simulink model "mainV02_12"  (R2016b)
settings: Solver=ode23s  StartTime=0.0  StopTime=inf  MaxStep=0.2  RelTol=1e-2
undefined symbols (not defined in the file): checks, deltae_degrees, deltafl_degrees, deltafr_degrees, deltar_degrees, deltat_1, deltat_2, deltat_3, deltat_4, deltat_5, Earth, F, ft, groundReaction, initialValues, LD, Light, m, MIL, Newton, Raphson, s, WGS84
libraries: aerolibutil x8, aerolibasang x5, aerolib6dof2 x4, aerolibwind2 x3, aerolibtransform2 x3, aerolib6dofsys x3, aerolibbdyn x3, aerolibconvert2 x3, aerolibconvert x2, aerolibatmos2 x1, aerolibobsolete x1, aerolibadyn x1
(part 1 of 3)
settings Model: Creator=Uxío  LastModifiedBy=sork9
settings DataIOCC: ReturnWorkspaceOutputs=on  ReturnWorkspaceOutputsName=spidata
settings OptimizationCC: EfficientMapNaN2IntZero=off  SimCompilerOptimization=on
settings DebuggingCC: ReadBeforeWriteMsg=DisableAll  WriteAfterWriteMsg=DisableAll  WriteAfterReadMsg=DisableAll  MultiTaskDSMMsg=none
settings HardwareCC: TargetBitPerPointer=64  TargetBitPerSizeT=64  TargetBitPerPtrDiffT=64  TargetLongLongMode=on  TargetIntDivRoundTo=Zero  TargetEndianess=LittleEndian  TargetWordSize=64  TargetHWDeviceType=MATLAB Host  ProdEqTarget=off
settings ModelReferenceCC: UpdateModelReferenceTargets=IfOutOfDate
settings SFSimCC: SFSimEcho=off
settings CodeAppCC: MaxIdLength=128
settings GRTTargetCC: TargetLangStandard=C89/C90 (ANSI)  CombineOutputUpdateFcns=off  GRTInterface=on
settings ConfigComp: PSAutoStubLUT=on

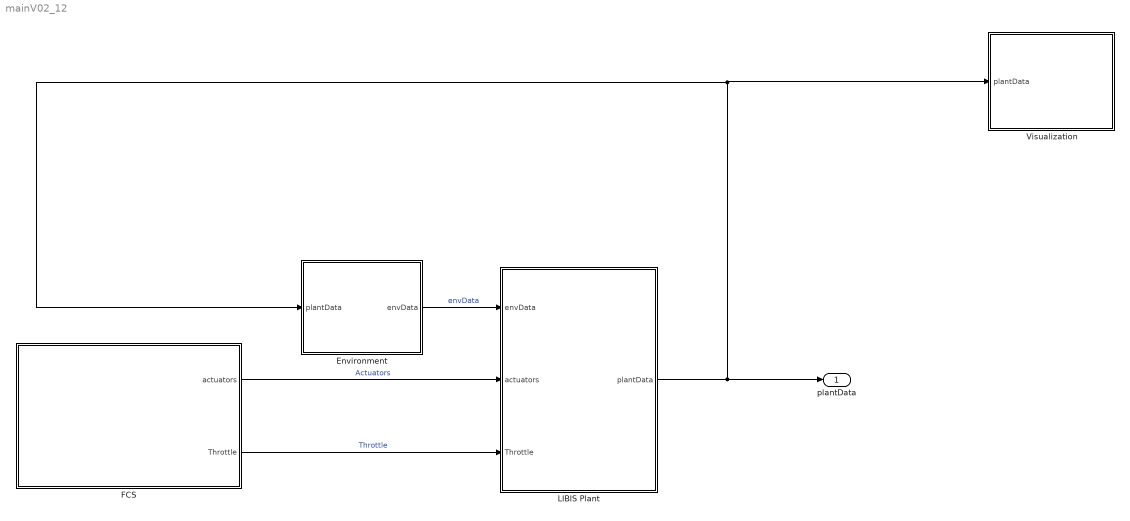
== system mainV02_12 ==
  Environment : Subsystem
      mask Display:
      | imageName='Wind.png';
      | currentPath=get_param(bdroot, 'FileName');
      | positions=strfind(currentPath,'\');
      | imagePath=strcat(currentPath(1:positions(end-1)),'graphics\',imageName);
      | image(imagePath);
  FCS : Subsystem
      mask Display:
      | imageName='FCS.png';
      | currentPath=get_param(bdroot, 'FileName');
      | positions=strfind(currentPath,'\');
      | imagePath=strcat(currentPath(1:positions(end-1)),'graphics\',imageName);
      | image(imagePath);
  LIBIS Plant : Subsystem
      mask Display:
      | imageName='LIBIS_Plant.jpg';
      | currentPath=get_param(bdroot, 'FileName');
      | positions=strfind(currentPath,'\');
      | imagePath=strcat(currentPath(1:positions(end-1)),'graphics\',imageName);
      | image(imagePath);
  Visualization : Subsystem
  plantData : Outport
  wires:
  Environment/1(envData) -> LIBIS Plant/1(envData)  "envData"
  FCS/1(actuators) -> LIBIS Plant/2(actuators)  "Actuators"
  FCS/2(Throttle) -> LIBIS Plant/3(Throttle)  "Throttle"
  LIBIS Plant/1(plantData) -> Environment/1(plantData), Visualization/1(plantData), plantData/1

== system mainV02_12/Environment ==
  plantData : Inport
  Bus Selector : BusSelector  OutputSignals=LLA.Altitude_m,X_ned,V_ned,DCM_body_earth,LLA.Latitude_deg
  COESA Atmosphere Model : aerolibatmos2/COESA Atmosphere Model  units=Metric (MKS)  spec=1976 COESA-extended U.S. Standard Atmosphere  model=Profile  profile_var=High temperature  profile_percent=1%  profile_alt=5 km (16404 ft)  envelope_var=High temperature  envelope_percent=1%  action=Warning
  Gravity in Earth Axes : Gain  Gain=[0 0 LD.Inertia.mass]  SaturateOnIntegerOverflow=on  OutDataTypeStr=Inherit: Same as input  ParamDataTypeStr=Inherit: Same as input
  Math Function : Math  Operator=transpose  SaturateOnIntegerOverflow=on
  Reshape : Reshape
  Reshape1 : Reshape
  Terrain : Subsystem
  To Body Axes : Product  Multiplication=Matrix(*)  SaturateOnIntegerOverflow=on  InputSameDT=on  OutDataTypeStr=Inherit: Same as first input
  To Body Axes1 : Product  Multiplication=Matrix(*)  SaturateOnIntegerOverflow=on  InputSameDT=on  OutDataTypeStr=Inherit: Same as first input
  WGS84 Gravity Model : aerolibobsolete/WGS84 Gravity Model  model=WGS84 Taylor Series  units=Metric (MKS)  no_atmos=on  precessing=on  month=February  day=1  year=2000  no_centrifugal=on  action=Warning
  Wind Models : Subsystem
  envDataBus : BusCreator  Inputs='h_ground','Fground','windVelocity','windOmega','T','a','P','AirDensity','Fgravity'  OutDataTypeStr=Bus: envDataBus  NonVirtualBus=on
  envData : Outport  InitialOutput=0
  wires:
  [Altitude] -> COESA Atmosphere Model/1
  Bus Selector/4 -> To Body Axes/1, Wind Models/3(DCM_be), To Body Axes1/1  "<DCM_body_earth>"
  Bus Selector/5 -> WGS84 Gravity Model/2  "<Latitude_deg>"
  Bus Selector/3 -> Wind Models/1(Ve), Terrain/2(Ve)  "<V_ned>"
  [Altitude] -> WGS84 Gravity Model/1
  envDataBus/1 -> envData/1  "envData"
  To Body Axes/1 -> Reshape/1  "Fg"
  Wind Models/2(windOmega) -> envDataBus/4  "windOmega"
  Bus Selector/2 -> Terrain/1(Xe)  "<X_ned>"
  WGS84 Gravity Model/1 -> Gravity in Earth Axes/1
  COESA Atmosphere Model/3 -> envDataBus/7  "P"
  COESA Atmosphere Model/2 -> envDataBus/6  "a"
  Wind Models/1(windVelocity) -> envDataBus/3  "windVelocity"
  [Altitude] -> Wind Models/2(Altitude)
  COESA Atmosphere Model/1 -> envDataBus/5  "T"
  COESA Atmosphere Model/4 -> envDataBus/8  "AirDensity"
  Terrain/1(hground) -> envDataBus/1  "h_ground"
  Bus Selector/1 -> [Altitude]  "<Altitude_m>"
  Gravity in Earth Axes/1 -> Math Function/1
  Math Function/1 -> To Body Axes/2
  Reshape/1 -> envDataBus/9  "Fgravity"
  To Body Axes1/1 -> Reshape1/1  "Fground_body"
  Reshape1/1 -> envDataBus/2  "Fground"
  Terrain/2(Fground) -> To Body Axes1/2  "Fground_earth"
  plantData/1 -> Bus Selector/1

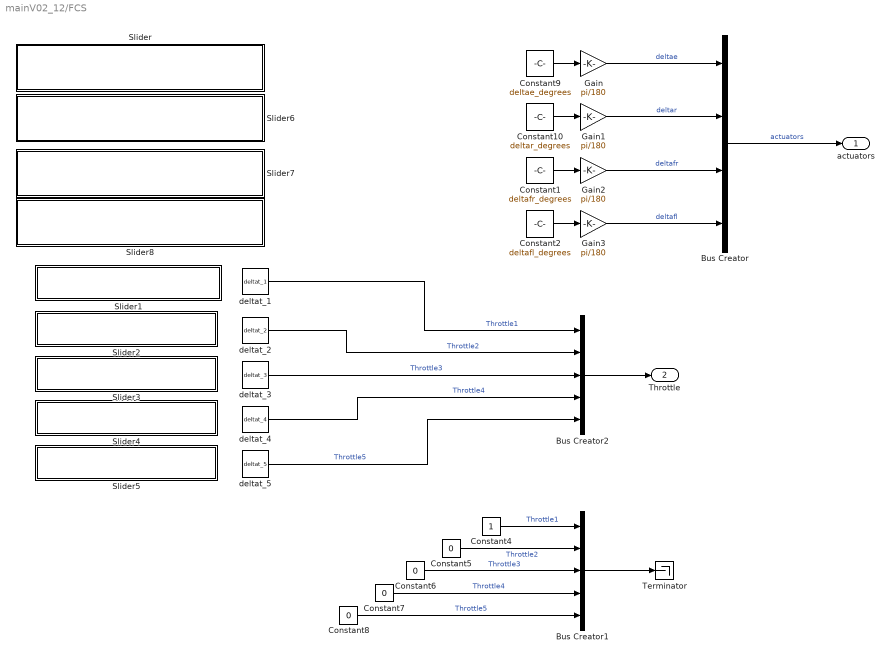
== system mainV02_12/FCS ==
  Bus Creator : BusCreator  Inputs=4
  Bus Creator1 : BusCreator  Inputs=5
  Bus Creator2 : BusCreator  Inputs=5
  Constant1 : Constant  Value=deltafr_degrees
  Constant10 : Constant  Value=deltar_degrees
  Constant2 : Constant  Value=deltafl_degrees
  Constant4 : Constant
  Constant{5..8} (4 alike) : Constant  Value=0
  Constant9 : Constant  Value=deltae_degrees
  Gain{,1..3} (4 alike) : Gain  Gain=pi/180
  Slider : Subsystem  DialogController=hmiCreateDDGDialog  IsWebBlock=on  mask(MWDashboardBlock){webBlockId=6273dd38-214f-4c77-9b1a-24b6ec7057c4, webBlockType=slider, ShowInLibBrowser=on, ShowInitialText=on, HMISrcModelName=mainV02_12}
      mask prompts: webBlockId "WebBlock Id"; webBlockType "WebBlock Type"; HMISrcModelName "Source Model"
      mask help: SimulinkHMI:dialogs:SliderDialogDesc
      mask Help: helpview([docroot '/mapfiles/simulink.map'], 'hmi_slider')
      mask Display:
      | if strcmp(get_param(bdroot(gcb),'BlockDiagramType'), 'library')
      |     image([(matlabroot) '/toolbox/simulink/hmi/icons/Slider.png']);
      | end
  Slider1 : Subsystem  DialogController=hmiCreateDDGDialog  IsWebBlock=on  mask(MWDashboardBlock){webBlockId=70020a0d-53bd-4fc8-9fe2-57375c6f10bc, webBlockType=slider, ShowInLibBrowser=on, ShowInitialText=on, HMISrcModelName=mainV02_12}
      mask prompts: webBlockId "WebBlock Id"; webBlockType "WebBlock Type"; HMISrcModelName "Source Model"
      mask help: SimulinkHMI:dialogs:SliderDialogDesc
      mask Help: helpview([docroot '/mapfiles/simulink.map'], 'hmi_slider')
      mask Display:
      | if strcmp(get_param(bdroot(gcb),'BlockDiagramType'), 'library')
      |     image([(matlabroot) '/toolbox/simulink/hmi/icons/Slider.png']);
      | end
  Slider2 : Subsystem  DialogController=hmiCreateDDGDialog  IsWebBlock=on  mask(MWDashboardBlock){webBlockId=1c2f52ab-856d-4c73-8b77-5cca8dc888a8, webBlockType=slider, ShowInLibBrowser=on, ShowInitialText=on, HMISrcModelName=mainV02_12}
      mask prompts: webBlockId "WebBlock Id"; webBlockType "WebBlock Type"; HMISrcModelName "Source Model"
      mask help: SimulinkHMI:dialogs:SliderDialogDesc
      mask Help: helpview([docroot '/mapfiles/simulink.map'], 'hmi_slider')
      mask Display:
      | if strcmp(get_param(bdroot(gcb),'BlockDiagramType'), 'library')
      |     image([(matlabroot) '/toolbox/simulink/hmi/icons/Slider.png']);
      | end
  Slider3 : Subsystem  DialogController=hmiCreateDDGDialog  IsWebBlock=on  mask(MWDashboardBlock){webBlockId=06ca73c2-e5c3-419a-af4c-8301bb851811, webBlockType=slider, ShowInLibBrowser=on, ShowInitialText=on, HMISrcModelName=mainV02_12}
      mask prompts: webBlockId "WebBlock Id"; webBlockType "WebBlock Type"; HMISrcModelName "Source Model"
      mask help: SimulinkHMI:dialogs:SliderDialogDesc
      mask Help: helpview([docroot '/mapfiles/simulink.map'], 'hmi_slider')
      mask Display:
      | if strcmp(get_param(bdroot(gcb),'BlockDiagramType'), 'library')
      |     image([(matlabroot) '/toolbox/simulink/hmi/icons/Slider.png']);
      | end
  Slider4 : Subsystem  DialogController=hmiCreateDDGDialog  IsWebBlock=on  mask(MWDashboardBlock){webBlockId=0f1aa799-7d0b-4e65-9c98-585766d84b05, webBlockType=slider, ShowInLibBrowser=on, ShowInitialText=on, HMISrcModelName=mainV02_12}
      mask prompts: webBlockId "WebBlock Id"; webBlockType "WebBlock Type"; HMISrcModelName "Source Model"
      mask help: SimulinkHMI:dialogs:SliderDialogDesc
      mask Help: helpview([docroot '/mapfiles/simulink.map'], 'hmi_slider')
      mask Display:
      | if strcmp(get_param(bdroot(gcb),'BlockDiagramType'), 'library')
      |     image([(matlabroot) '/toolbox/simulink/hmi/icons/Slider.png']);
      | end
  Slider5 : Subsystem  DialogController=hmiCreateDDGDialog  IsWebBlock=on  mask(MWDashboardBlock){webBlockId=1aba3140-aa7a-42dc-9545-4aab801dd215, webBlockType=slider, ShowInLibBrowser=on, ShowInitialText=on, HMISrcModelName=mainV02_12}
      mask prompts: webBlockId "WebBlock Id"; webBlockType "WebBlock Type"; HMISrcModelName "Source Model"
      mask help: SimulinkHMI:dialogs:SliderDialogDesc
      mask Help: helpview([docroot '/mapfiles/simulink.map'], 'hmi_slider')
      mask Display:
      | if strcmp(get_param(bdroot(gcb),'BlockDiagramType'), 'library')
      |     image([(matlabroot) '/toolbox/simulink/hmi/icons/Slider.png']);
      | end
  Slider6 : Subsystem  DialogController=hmiCreateDDGDialog  IsWebBlock=on  mask(MWDashboardBlock){webBlockId=3d9f47b7-f15d-42be-b3f0-4bf7c2d4a508, webBlockType=slider, ShowInLibBrowser=on, ShowInitialText=on, HMISrcModelName=mainV02_12}
      mask prompts: webBlockId "WebBlock Id"; webBlockType "WebBlock Type"; HMISrcModelName "Source Model"
      mask help: SimulinkHMI:dialogs:SliderDialogDesc
      mask Help: helpview([docroot '/mapfiles/simulink.map'], 'hmi_slider')
      mask Display:
      | if strcmp(get_param(bdroot(gcb),'BlockDiagramType'), 'library')
      |     image([(matlabroot) '/toolbox/simulink/hmi/icons/Slider.png']);
      | end
  Slider7 : Subsystem  DialogController=hmiCreateDDGDialog  IsWebBlock=on  mask(MWDashboardBlock){webBlockId=8e5c7658-11f4-4f70-8154-234cc52576e8, webBlockType=slider, ShowInLibBrowser=on, ShowInitialText=on, HMISrcModelName=mainV02_12}
      mask prompts: webBlockId "WebBlock Id"; webBlockType "WebBlock Type"; HMISrcModelName "Source Model"
      mask help: SimulinkHMI:dialogs:SliderDialogDesc
      mask Help: helpview([docroot '/mapfiles/simulink.map'], 'hmi_slider')
      mask Display:
      | if strcmp(get_param(bdroot(gcb),'BlockDiagramType'), 'library')
      |     image([(matlabroot) '/toolbox/simulink/hmi/icons/Slider.png']);
      | end
  Slider8 : Subsystem  DialogController=hmiCreateDDGDialog  IsWebBlock=on  mask(MWDashboardBlock){webBlockId=fd4f6454-3dcd-4a0d-9f3e-71aa520b8d15, webBlockType=slider, ShowInLibBrowser=on, ShowInitialText=on, HMISrcModelName=mainV02_12}
      mask prompts: webBlockId "WebBlock Id"; webBlockType "WebBlock Type"; HMISrcModelName "Source Model"
      mask help: SimulinkHMI:dialogs:SliderDialogDesc
      mask Help: helpview([docroot '/mapfiles/simulink.map'], 'hmi_slider')
      mask Display:
      | if strcmp(get_param(bdroot(gcb),'BlockDiagramType'), 'library')
      |     image([(matlabroot) '/toolbox/simulink/hmi/icons/Slider.png']);
      | end
  Terminator : Terminator
  deltat_1 : Constant  Value=deltat_1
  deltat_2 : Constant  Value=deltat_2
  deltat_3 : Constant  Value=deltat_3
  deltat_4 : Constant  Value=deltat_4
  deltat_5 : Constant  Value=deltat_5
  actuators : Outport
  Throttle : Outport  Port=2
  wires:
  Bus Creator/1 -> actuators/1  "actuators"
  Gain1/1 -> Bus Creator/2  "deltar"
  Gain2/1 -> Bus Creator/3  "deltafr"
  Gain3/1 -> Bus Creator/4  "deltafl"
  Constant4/1 -> Bus Creator1/1  "Throttle1"
  Constant5/1 -> Bus Creator1/2  "Throttle2"
  Constant6/1 -> Bus Creator1/3  "Throttle3"
  Constant7/1 -> Bus Creator1/4  "Throttle4"
  Constant8/1 -> Bus Creator1/5  "Throttle5"
  Gain/1 -> Bus Creator/1  "deltae"
  Constant9/1 -> Gain/1
  deltat_1/1 -> Bus Creator2/1  "Throttle1"
  deltat_3/1 -> Bus Creator2/3  "Throttle3"
  deltat_2/1 -> Bus Creator2/2  "Throttle2"
  Bus Creator2/1 -> Throttle/1
  deltat_4/1 -> Bus Creator2/4  "Throttle4"
  deltat_5/1 -> Bus Creator2/5  "Throttle5"
  Bus Creator1/1 -> Terminator/1
  Constant10/1 -> Gain1/1
  Constant1/1 -> Gain2/1
  Constant2/1 -> Gain3/1

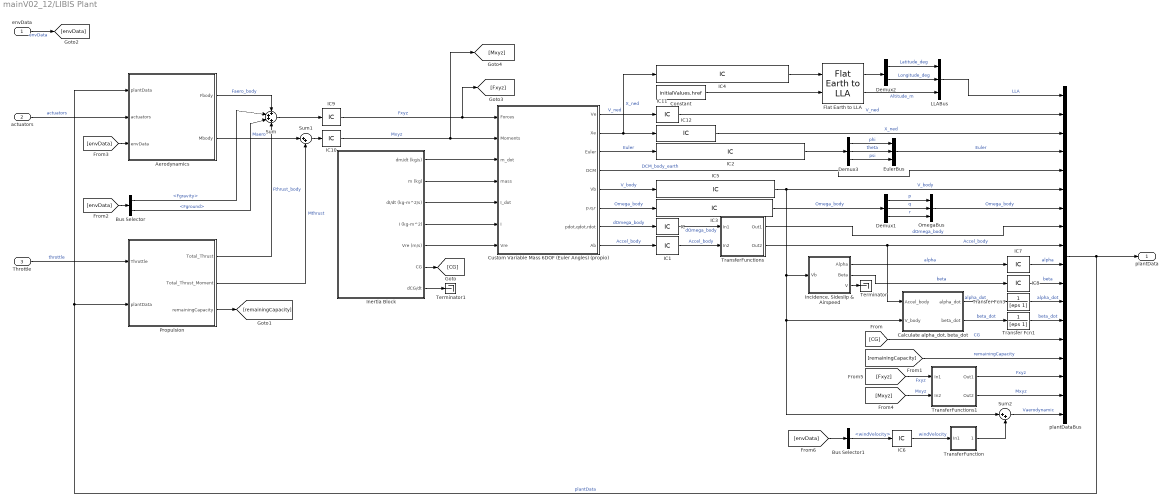
== system mainV02_12/LIBIS Plant ==
  envData : Inport
  actuators : Inport  Port=2
  Throttle : Inport  Port=3
  Aerodynamics : Subsystem
  Bus Selector : BusSelector  OutputSignals=Fgravity,Fground
  Bus Selector1 : BusSelector  OutputSignals=windVelocity
  "Calculate alpha_dot, beta_dot" : Subsystem
  Constant : Constant  Value=initialValues.href
  Custom Variable Mass 6DOF (Euler Angles) (propio) : Subsystem  mask(6DOF EoM (Body Axis)){units=Metric (MKS), mtype=Custom Variable, rep=Euler Angles, xme_0=[initialValues.Xe0 initialValues.Ye0 initialValues.Ze0], Vm_0=[initialValues.u0 initialValues.v0 initialValues.w0], eul_0=[initialValues.roll0 initialValues.pitch0 initialValues.yaw0], pm_0=[initialValues.p0 initialValues.q0 initialValues.r0], mass_0=1.0, mass_e=0.5, mass_f=2.0, inertia=eye(3), inertia_e=eye(3), inertia_f=2*eye(3), k_quat=1.0, vre_flag=on}
      mask prompts: units "aeroblks:aeroblk6dofbody:block6DOFEoMBodyAxisParamUnits"; mtype "aeroblks:aeroblk6dofbody:block6DOFEoMBodyAxisParamMasstype"; rep "aeroblks:aeroblk6dofbody:block6DOFEoMBodyAxisParamRepresentation"; xme_0 "aeroblks:aeroblk6dofbody:block6DOFEoMBodyAxisParamInitialpositionininertialaxesXeYeZe"; Vm_0 "aeroblks:aeroblk6dofbody:block6DOFEoMBodyAxisParamInitialvelocityinbodyaxesUvw"; eul_0 "aeroblks:aeroblk6dofbody:block6DOFEoMBodyAxisParamInitialEulerorientationrollpitchyaw"; pm_0 "aeroblks:aeroblk6dofbody:block6DOFEoMBodyAxisParamInitialbodyrotationratespqr"; mass_0 "aeroblks:aeroblk6dofbody:block6DOFEoMBodyAxisParamInitialmass"; mass_e "aeroblks:aeroblk6dofbody:block6DOFEoMBodyAxisParamEmptymass"; mass_f "aeroblks:aeroblk6dofbody:block6DOFEoMBodyAxisParamFullmass"; inertia "aeroblks:aeroblk6dofbody:block6DOFEoMBodyAxisParamInertia"; inertia_e "aeroblks:aeroblk6dofbody:block6DOFEoMBodyAxisParamEmptyinertiamatrix"; inertia_f "aeroblks:aeroblk6dofbody:block6DOFEoMBodyAxisParamFullinertiamatrix"; k_quat "aeroblks:aeroblk6dofbody:block6DOFEoMBodyAxisParamGainforquaternionnormalization"; vre_flag "aeroblks:aeroblk6dofbody:block6DOFEoMBodyAxisParamIncludemassflowrelativevelocity"
      mask help: aeroblks:aeroblk6dofbody:block6DOFEoMBodyAxisDesc
      mask init:
      | ports=aeroicon('aeroblk6dofbody','icon');
      mask Help: eval('asbhelp(''custom_variable_mass_sixdof_euler_angles'')');
      mask TypeOptions units: aeroblks:aeroblk6dofbody:block6DOFEoMBodyAxisParamComboMetricMKS | aeroblks:aeroblk6dofbody:block6DOFEoMBodyAxisParamComboEnglishVelocityinfts | aeroblks:aeroblk6dofbody:block6DOFEoMBodyAxisParamComboEnglishVelocityinkts
      mask TypeOptions mtype: aeroblks:aeroblk6dofbody:block6DOFEoMBodyAxisParamComboFixed | aeroblks:aeroblk6dofbody:block6DOFEoMBodyAxisParamComboSimpleVariable | aeroblks:aeroblk6dofbody:block6DOFEoMBodyAxisParamComboCustomVariable
      mask Callback mtype: aeroicon('aeroblk6dofbody');
      mask TypeOptions rep: aeroblks:aeroblk6dofbody:block6DOFEoMBodyAxisParamComboEulerAngles | aeroblks:aeroblk6dofbody:block6DOFEoMBodyAxisParamComboQuaternion
      mask Callback rep: aeroicon('aeroblk6dofbody');
      mask Display:
      | port_label(ports(1).type,ports(1).port,ports(1).txt,'texmode','on');
      | port_label(ports(2).type,ports(2).port,ports(2).txt,'texmode','on');
      | port_label(ports(3).type,ports(3).port,ports(3).txt,'texmode','on');
      | port_label(ports(4).type,ports(4).port,ports(4).txt,'texmode','on');
      | port_label(ports(5).type,ports(5).port,ports(5).txt,'texmode','on');
      | port_label(ports(6).type,ports(6).port,ports(6).txt,'texmode','on');
      | port_label(ports(7).type,ports(7).port,ports(7).txt,'texmode','on');
      | port_label(ports(8).type,ports(8).port,ports(8).txt,'texmode','on');
      | port_label(ports(9).type,ports(9).port,ports(9).txt,'texmode','on');
      | port_label(ports(10).type,ports(10).port,ports(10).txt,'texmode','on');
      | port_label(ports(11).type,ports(11).port,ports(11).txt,'texmode','on');
      | port_label(ports(12).type,ports(12).port,ports(12).txt,'texmode','on');
      | port_label(ports(13).type,ports(13).port,ports(13).txt,'texmode','on');
      | port_label(ports(14).type,ports(14).port,ports(14).txt,'texmode','on');
      | port_label(ports(15).type,ports(15).port,ports(15).txt,'texmode','on');
      | port_label(ports(16).type,ports(16).port,ports(16).txt,'texmode','on');
      | [x y xp yp highstr lowstr maxy miny]=aeroimage('sixdofbody',gcbh);
      | text(0.5,maxy+0.065,highstr{:},'horizontalAlignment','center')
      | text(0.5,miny-0.06,lowstr{:},'horizontalAlignment','center')
      | plot(x,y);
      | patch(xp, yp);
  Demux1 : Demux  Outputs=3
  Demux2 : Demux  Outputs=2
  Demux3 : Demux  Outputs=3
  EulerBus : BusCreator  Inputs='phi','theta','psi'  OutDataTypeStr=Bus: EulerBus  NonVirtualBus=on
  Flat Earth to LLA : aerolibtransform2/Flat Earth to LLA  units=Metric (MKS)  ptype=Earth (WGS84)  F=1/298.257223563  R=6378137  LL0=initialValues.LatLong0  psi=initialValues.heading0
  IC{,1,6,9..11} (6 alike) : InitialCondition  Value=[0 0 0]
  IC12 : InitialCondition  Value=[0 0 -initialValues.href]
  IC2 : InitialCondition  Value=[initialValues.roll0, initialValues.pitch0, initialValues.yaw0]
  IC3 : InitialCondition  Value=[initialValues.p0 initialValues.q0 initialValues.r0]
  IC4 : InitialCondition  Value=[initialValues.Xe0 initialValues.Ye0 initialValues.Ze0]
  IC5 : InitialCondition  Value=[initialValues.u0 initialValues.v0 initialValues.w0]
  IC7 : InitialCondition  Value=0
  IC8 : InitialCondition  Value=0
  "Incidence, Sideslip & Airspeed" : Subsystem
  Inertia Block : Subsystem
      mask Display:
      | imageName='Moment_of_inertia.png';
      | currentPath=get_param(bdroot, 'FileName');
      | positions=strfind(currentPath,'\');
      | imagePath=strcat(currentPath(1:positions(end-1)),'graphics\',imageName);
      | image(imagePath);
  LLABus : BusCreator  Inputs='Latitude_deg','Longitude_deg','Altitude_m'  OutDataTypeStr=Bus: LLABus  NonVirtualBus=on
  OmegaBus : BusCreator  Inputs='p','q','r'  OutDataTypeStr=Bus: OmegaBus  NonVirtualBus=on
  Propulsion : Subsystem
  Sum : Sum  Inputs=++++
  Sum1 : Sum  Inputs=|++
  Sum2 : Sum  Inputs=|++
  Terminator : Terminator
  Terminator1 : Terminator
  Transfer Fcn1 : TransferFcn  Denominator=[eps 1]
  Transfer Fcn3 : TransferFcn  Denominator=[eps 1]
  TransferFunction : Subsystem
  TransferFunctions : Subsystem
  TransferFunctions1 : Subsystem
  plantDataBus : BusCreator  Inputs='LLA','V_ned','X_ned','Euler','DCM_body_earth','V_body','Omega_body','dOmega_body','Accel_body','alpha','beta','alpha_dot','beta_dot','CG','remainingCapacity','Fxyz','Mxyz','Vaerodynamic'  OutDataTypeStr=Bus: plantDataBus  NonVirtualBus=on
  plantData : Outport
  wires:
  Inertia Block/4(I (kg-m^2)) -> Custom Variable Mass 6DOF (Euler Angles) (propio)/6(I)
  plantDataBus/1 -> Propulsion/2(plantData), Aerodynamics/1(plantData), plantData/1  "plantData"
  Flat Earth to LLA/2 -> LLABus/3  "Altitude_m"
  Custom Variable Mass 6DOF (Euler Angles) (propio)/2(Xe) -> IC12/1, IC4/1  "X_ned"
  "Incidence, Sideslip & Airspeed"/3(V) -> Terminator/1
  Custom Variable Mass 6DOF (Euler Angles) (propio)/3(Euler) -> IC2/1  "Euler"
  EulerBus/1 -> plantDataBus/4  "Euler"
  Flat Earth to LLA/1 -> Demux2/1
  Demux2/1 -> LLABus/1  "Latitude_deg"
  Inertia Block/2(m (kg)) -> Custom Variable Mass 6DOF (Euler Angles) (propio)/4(mass)
  Inertia Block/5(Vre (m/s)) -> Custom Variable Mass 6DOF (Euler Angles) (propio)/7(Vre)
  Custom Variable Mass 6DOF (Euler Angles) (propio)/5(Vb) -> IC5/1  "V_body"
  Inertia Block/7(dCG/dt) -> Terminator1/1
  [CG] -> plantDataBus/14  "CG"
  Custom Variable Mass 6DOF (Euler Angles) (propio)/4(DCM) -> plantDataBus/5  "DCM_body_earth"
  Inertia Block/3(dI/dt (kg-m^2/s)) -> Custom Variable Mass 6DOF (Euler Angles) (propio)/5(I_dot)
  LLABus/1 -> plantDataBus/1  "LLA"
  "Incidence, Sideslip & Airspeed"/1(Alpha) -> IC7/1  "alpha"
  Demux3/1 -> EulerBus/1  "phi"
  Demux3/3 -> EulerBus/3  "psi"
  Inertia Block/6(CG) -> [CG]
  Inertia Block/1(dm/dt (kg/s)) -> Custom Variable Mass 6DOF (Euler Angles) (propio)/3(m_dot)
  Constant/1 -> Flat Earth to LLA/2
  Demux2/2 -> LLABus/2  "Longitude_deg"
  "Incidence, Sideslip & Airspeed"/2(Beta) -> IC8/1  "beta"
  Demux3/2 -> EulerBus/2  "theta"
  Custom Variable Mass 6DOF (Euler Angles) (propio)/1(Ve) -> IC11/1  "V_ned"
  OmegaBus/1 -> plantDataBus/7  "Omega_body"
  Custom Variable Mass 6DOF (Euler Angles) (propio)/6(p,q,r) -> IC3/1  "Omega_body"
  Demux1/2 -> OmegaBus/2  "q"
  Demux1/1 -> OmegaBus/1  "p"
  Demux1/3 -> OmegaBus/3  "r"
  Propulsion/2(Total_Thrust_Moment) -> Sum1/2  "Mthrust"
  actuators/1 -> Aerodynamics/2(actuators)  "actuators"
  Throttle/1 -> Propulsion/1(Throttle)  "throttle"
  Propulsion/3(remainingCapacity) -> [remainingCapacity]
  [remainingCapacity] -> plantDataBus/15  "remainingCapacity"
  Propulsion/1(Total_Thrust) -> Sum/4  "Fthrust_body"
  envData/1 -> [envData]  "envData"
  [envData] -> Bus Selector/1
  [envData] -> Aerodynamics/3(envData)
  IC4/1 -> Flat Earth to LLA/1
  IC5/1 -> plantDataBus/6, "Incidence, Sideslip & Airspeed"/1(Vb), Sum2/1, "Calculate alpha_dot, beta_dot"/2(V_body)  "V_body"
  IC3/1 -> Demux1/1  "Omega_body"
  Aerodynamics/1(Fbody) -> Sum/1  "Faero_body"
  Aerodynamics/2(Mbody) -> Sum1/1  "Maero"
  IC2/1 -> Demux3/1
  Bus Selector/1 -> Sum/2  "<Fgravity>"
  IC7/1 -> plantDataBus/10  "alpha"
  "Calculate alpha_dot, beta_dot"/1(alpha_dot) -> Transfer Fcn3/1  "alpha_dot"
  "Calculate alpha_dot, beta_dot"/2(beta_dot) -> Transfer Fcn1/1  "beta_dot"
  [envData] -> Bus Selector1/1
  Bus Selector/2 -> Sum/3  "<Fground>"
  Bus Selector1/1 -> IC6/1  "<windVelocity>"
  Sum2/1 -> plantDataBus/18  "Vaerodynamic"
  Custom Variable Mass 6DOF (Euler Angles) (propio)/7(pdot,qdot,rdot) -> IC/1  "dOmega_body"
  Custom Variable Mass 6DOF (Euler Angles) (propio)/8(Ab) -> IC1/1  "Accel_body"
  IC8/1 -> plantDataBus/11  "beta"
  IC6/1 -> TransferFunction/1(In1)  "windVelocity"
  Sum1/1 -> IC10/1
  Sum/1 -> IC9/1
  IC9/1 -> [Fxyz], Custom Variable Mass 6DOF (Euler Angles) (propio)/1(Forces)  "Fxyz"
  IC10/1 -> [Mxyz], Custom Variable Mass 6DOF (Euler Angles) (propio)/2(Moments)  "Mxyz"
  IC/1 -> TransferFunctions/1(In1)  "dOmega_body"
  IC1/1 -> TransferFunctions/2(In2)  "Accel_body"
  TransferFunctions/1(Out1) -> plantDataBus/8  "dOmega_body"
  TransferFunctions/2(Out2) -> plantDataBus/9, "Calculate alpha_dot, beta_dot"/1(Accel_body)  "Accel_body"
  IC11/1 -> plantDataBus/2  "V_ned"
  IC12/1 -> plantDataBus/3  "X_ned"
  Transfer Fcn3/1 -> plantDataBus/12  "alpha_dot"
  TransferFunction/1(Out1) -> Sum2/2
  Transfer Fcn1/1 -> plantDataBus/13  "beta_dot"
  [Mxyz] -> TransferFunctions1/2(In2)  "Mxyz"
  [Fxyz] -> TransferFunctions1/1(In1)  "Fxyz"
  TransferFunctions1/1(Out1) -> plantDataBus/16  "Fxyz"
  TransferFunctions1/2(Out2) -> plantDataBus/17  "Mxyz"

== system mainV02_12/Visualization ==
  plantData : Inport
  Airspeed Indicator : Subsystem  DialogController=aeroblksHMICreateDDGDialog  IsWebBlock=on  mask(MWDashboardBlock){webBlockId=1660c180-4922-4edc-b12a-b6c4fb3472e7, webBlockType=airspeedindicator, ShowInLibBrowser=on, ShowInitialText=on, HMISrcModelName=mainV02_12}
      mask prompts: webBlockId "WebBlock Id"; webBlockType "WebBlock Type"; HMISrcModelName "Source Model"
      mask help: aeroblksHMI:aeroblkhmi:AirspeedIndicatorDialogDesc
      mask Help: eval('asbhmihelp(''airspeedindicator'')');
      mask Display:
      | if strcmp(get_param(bdroot(gcb),'BlockDiagramType'), 'library')
      |  image([(matlabroot) '/toolbox/aeroblks/aeroblks/hmi/icons/AirspeedIndicatorIcon.svg'])
      | end
  Alpha and beta visualization : Scope  NumInputPorts=2
  Altimeter : Subsystem  DialogController=aeroblksHMICreateDDGDialog  IsWebBlock=on  mask(MWDashboardBlock){webBlockId=dac4b64b-8b08-4b88-951c-85bcef5f9a8d, webBlockType=altimeter, ShowInLibBrowser=on, ShowInitialText=on, HMISrcModelName=mainV02_12}
      mask prompts: webBlockId "WebBlock Id"; webBlockType "WebBlock Type"; HMISrcModelName "Source Model"
      mask help: aeroblksHMI:aeroblkhmi:AltimeterDialogDesc
      mask Help: eval('asbhmihelp(''altimeter'')');
      mask Display:
      | if strcmp(get_param(bdroot(gcb),'BlockDiagramType'), 'library')
      |  image([(matlabroot) '/toolbox/aeroblks/aeroblks/hmi/icons/AltimeterIcon.svg'])
      | end
  Altitude : Scope
  Artificial Horizon : Subsystem  DialogController=aeroblksHMICreateDDGDialog  IsWebBlock=on  mask(MWDashboardBlock){webBlockId=71b89583-386f-4e5a-a87e-fbc6faf0c9b0, webBlockType=artificialhorizon, ShowInLibBrowser=on, ShowInitialText=on, HMISrcModelName=mainV02_12}
      mask prompts: webBlockId "WebBlock Id"; webBlockType "WebBlock Type"; HMISrcModelName "Source Model"
      mask help: aeroblksHMI:aeroblkhmi:ArtificialHorizonDialogDesc
      mask Help: eval('asbhmihelp(''artificialhorizon'')');
      mask Display:
      | if strcmp(get_param(bdroot(gcb),'BlockDiagramType'), 'library')
      |  image([(matlabroot) '/toolbox/aeroblks/aeroblks/hmi/icons/ArtificialHorizonIcon.svg'])
      | end
  Axes to VR Axes : Subsystem
  Bus Selector : BusSelector  OutputSignals=X_ned
  Bus Selector1 : BusSelector  OutputSignals=Euler.phi,Euler.theta,Euler.psi
  Bus Selector2 : BusSelector  OutputSignals=LLA.Altitude_m
  Bus Selector3 : BusSelector  OutputSignals=V_body,V_ned
  Bus Selector4 : BusSelector  OutputSignals=alpha,beta
  Climb Rate Indicator : Subsystem  DialogController=aeroblksHMICreateDDGDialog  IsWebBlock=on  mask(MWDashboardBlock){webBlockId=2290786a-142e-4cdc-9e89-cbe88d1b2ef4, webBlockType=climbindicator, ShowInLibBrowser=on, ShowInitialText=on, HMISrcModelName=mainV02_12}
      mask prompts: webBlockId "WebBlock Id"; webBlockType "WebBlock Type"; HMISrcModelName "Source Model"
      mask help: aeroblksHMI:aeroblkhmi:ClimbIndicatorDialogDesc
      mask Help: eval('asbhmihelp(''climbindicator'')');
      mask Display:
      | if strcmp(get_param(bdroot(gcb),'BlockDiagramType'), 'library')
      |  image([(matlabroot) '/toolbox/aeroblks/aeroblks/hmi/icons/ClimbIndicatorIcon.svg'])
      | end
  Demux : Demux  Outputs=3
  Demux1 : Demux  Outputs=3
  Demux2 : Demux  Outputs=3
  Earth position : Scope  NumInputPorts=3
  Euler angles visualization : Scope  NumInputPorts=3
  Euler to VR : Subsystem
  Heading Indicator : Subsystem  DialogController=aeroblksHMICreateDDGDialog  IsWebBlock=on  mask(MWDashboardBlock){webBlockId=f0aafb45-9505-4aed-89ac-b6a93bae7c37, webBlockType=headingindicator, ShowInLibBrowser=on, ShowInitialText=on, HMISrcModelName=mainV02_12}
      mask prompts: webBlockId "WebBlock Id"; webBlockType "WebBlock Type"; HMISrcModelName "Source Model"
      mask help: aeroblksHMI:aeroblkhmi:HeadingIndicatorDialogDesc
      mask Help: eval('asbhmihelp(''headingindicator'')');
      mask Display:
      | if strcmp(get_param(bdroot(gcb),'BlockDiagramType'), 'library')
      |  image([(matlabroot) '/toolbox/aeroblks/aeroblks/hmi/icons/HeadingIndicatorIcon.svg'])
      | end
  Mux : Mux  Inputs=3
  Subsystem : Subsystem
  Terminator{,1..4} (5 alike) : Terminator
  VR Sink : vrlib/VR Sink  InstantiateOnLoad=on  SampleTime=0.1  ViewEnable=on  RemoteChange=off  RemoteView=off  FieldsWritten=HL20.rotation.4.1.1.double#HL20.translation.3.1.1.double  WorldFileName=aeroblk_HL20.wrl  WorldDescription=aeroblk_HL20  AutoView=on  VideoDimensions=[]  AllowVariableSize=off  FigureProperties="{'Position', 'Name', 'Viewpoint', 'CameraBound', 'CameraDirection', 'CameraPosition', 'CameraUpVector', 'ZoomFactor', 'Antialiasing', 'Headlight', 'Lighting', 'NavPanel', 'Sound', 'StatusBar', 'Stereo3D', 'Stereo3DCameraOffset', 'Stereo3DHIT', 'ToolBar', 'Textures', 'Transparency', 'Triad', 'Wireframe', 'NavZones', 'NavMode', 'NavSpeed', 'CaptureFileFormat', 'CaptureFileName', 'Record2DCompressMethod', 'Record2DCompressQuality', 'Record2D', 'Record2DFileName', 'Record2DFPS'; [1.9220000000000000e+03   8.4000000000000000e+01   6.8100000000000000e+02   5.9200000000000000e+02], 'aeroblk_HL20', 'Rear Position', 'on', [0.0000000000000000e+00   0.0000000000000000e+00  -1.0000000000000000e+00], [0.0000000000000000e+00   0.0000000000000000e+00   0.0000000000000000e+00], [0.0000000000000000e+00   1.0000000000000000e+00   0.0000000000000000e+00], [1.0000000000000000e+00], 'on', 'on', 'on', 'halfbar', 'on', 'on', 'off', [1.0000000149011612e-01], [0.0000000000000000e+00], 'on', 'on', 'on', 'none', 'off', 'off', 'fly', 'normal', 'tif', '%f_anim_%n.tif', 'auto', [7.5000000000000000e+01], 'off', '%f_anim_%n.avi', 'auto'}"
  V_body visualization : Scope  NumInputPorts=3
  V_ned visualization : Scope  NumInputPorts=3
  wires:
  Bus Selector1/1 -> Euler angles visualization/1, Mux/1  "<phi>"
  Bus Selector1/2 -> Mux/2, Euler angles visualization/2  "<theta>"
  Bus Selector1/3 -> Euler angles visualization/3, Mux/3  "<psi>"
  plantData/1 -> Bus Selector4/1, Bus Selector3/1, Bus Selector2/1, Bus Selector/1, Bus Selector1/1
  Bus Selector2/1 -> Altitude/1  "<Altitude_m>"
  Euler to VR/1(Axis Angle) -> VR Sink/1
  Axes to VR Axes/1(Xe VR) -> VR Sink/2
  Bus Selector/1 -> Demux/1, Axes to VR Axes/1(Xe), Subsystem/1("X_ned ")  "<X_ned>"
  Mux/1 -> Subsystem/2(Euler_angles), Euler to VR/1(Euler Angles)
  Bus Selector3/1 -> Demux2/1, Subsystem/3(V_body)  "<V_body>"
  Bus Selector3/2 -> Demux1/1, Subsystem/4(V_ned)  "<V_ned>"
  Subsystem/1(Airspeed (kts)) -> Terminator/1
  Subsystem/2(Height (ft)) -> Terminator1/1
  Subsystem/3(Roll Flightpath (deg)) -> Terminator2/1
  Subsystem/4(Climb Rate (ft/min)) -> Terminator3/1
  Subsystem/5(Heading (deg)) -> Terminator4/1
  Demux/2 -> Earth position/2
  Demux/1 -> Earth position/1
  Demux/3 -> Earth position/3
  Bus Selector4/1 -> Alpha and beta visualization/1  "<alpha>"
  Bus Selector4/2 -> Alpha and beta visualization/2  "<beta>"
  Demux1/1 -> V_ned visualization/1  "V_ned_x"
  Demux1/2 -> V_ned visualization/2  "V_ned_y"
  Demux1/3 -> V_ned visualization/3  "V_ned_z"
  Demux2/1 -> V_body visualization/1  "V_body_x"
  Demux2/2 -> V_body visualization/2  "V_body_y"
  Demux2/3 -> V_body visualization/3  "V_body_z"

== system mainV02_12/Environment/Terrain ==
  Xe : Inport  Unit=m
  Ve : Inport  Port=2
  -D : Gain  Gain=-groundReaction.D
  -K : Gain  Gain=-groundReaction.K
  -K1 : Gain  Gain=-groundReaction.Mu
  -K3 : Gain  Gain=-groundReaction.Mu
  Constant : Constant  Value=0
  Constant1 : Constant  Value=0
  Constant2 : Constant  Value=0
  Mux : Mux  Inputs=3
  Product : Product
  Sel1 : Selector  InputPortWidth=3  IndexOptions=Index vector (dialog)  Indices=3  OutputSizes=1
  Sel2 : Selector  InputPortWidth=3  IndexOptions=Index vector (dialog)  Indices=3  OutputSizes=1
  Sel3 : Selector  InputPortWidth=3  IndexOptions=Index vector (dialog)  Indices=1  OutputSizes=1
  Sel4 : Selector  InputPortWidth=3  IndexOptions=Index vector (dialog)  Indices=2  OutputSizes=1
  Sqrt : Sqrt  SaturateOnIntegerOverflow=on
  Sum : Sum  Inputs=|++
  Sum1 : Sum  Inputs=-+
  Switch : Switch  Criteria=u2 > Threshold
  Switch1 : Switch  Criteria=u2 > Threshold
  Switch2 : Switch  Criteria=u2 > Threshold
  Ze2height : UnaryMinus
  Ze_dot2height_dot : UnaryMinus
  Ze_dot2height_dot1 : UnaryMinus
  Ze_dot2height_dot2 : UnaryMinus
  height2d : UnaryMinus
  height2d1 : UnaryMinus
  hground_value : Constant  Value=initialValues.href  OutDataTypeStr=double
  hground : Outport  Unit=m
  Fground : Outport  Port=2  Unit=N
  wires:
  Xe/1 -> Sel2/1
  hground_value/1 -> Sum1/1
  Ze2height/1 -> Sum1/2  "alt"
  Sel2/1 -> Ze2height/1
  Sel1/1 -> Ze_dot2height_dot/1
  Constant/1 -> Switch/1
  Switch/1 -> height2d/1
  height2d/1 -> Sqrt/1  "d"
  Ze_dot2height_dot/1 -> -D/1  "z_dot"
  -K/1 -> Sum/1
  -D/1 -> Sum/2
  Sqrt/1 -> Product/1
  Sum/1 -> Product/2
  Product/1 -> height2d1/1
  Mux/1 -> Fground/1
  height2d1/1 -> Mux/3
  Sel3/1 -> Ze_dot2height_dot1/1
  Ze_dot2height_dot1/1 -> -K1/1
  Sel4/1 -> Ze_dot2height_dot2/1
  Ze_dot2height_dot2/1 -> -K3/1
  -K1/1 -> Switch1/3  "z"
  Sum1/1 -> Switch2/2, Switch1/2, hground/1, -K/1, Switch/3, Switch/2  "z"
  Constant1/1 -> Switch1/1
  Switch1/1 -> Mux/1
  Switch2/1 -> Mux/2
  Constant2/1 -> Switch2/1
  -K3/1 -> Switch2/3
  Ve/1 -> Sel3/1, Sel4/1, Sel1/1

== system mainV02_12/Environment/Wind Models ==
  Ve : Inport
  Altitude : Inport  Port=2
  DCM_be : Inport  Port=3
  Discrete Wind Gust Model : aerolibwind2/Discrete Wind Gust Model  units=Metric (MKS)  Gx=off  Gy=off  Gz=off  t_0=20  d_m=[120 120 80]  v_m=[3.5 3.0 3.0]
  Dot Product : DotProduct  OutDataTypeStr=Inherit: Inherit via internal rule
  Dryden Wind Turbulence Model (Continuous (+q +r)) : aerolibwind2/Dryden Wind Turbulence Model  (Continuous (+q -r))  units=Metric (MKS)  spec=MIL-F-8785C  model=Continuous Dryden (+q +r)  W20=5  Wdeg=0  TurbProb=10^-2 - Light  L_high=533.4  Wingspan=4  ts=0.1  Seed=[23341 23342 23343 23344]  T_on=off
  Sum : Sum  Inputs=+++  SaturateOnIntegerOverflow=on  InputSameDT=on  OutDataTypeStr=Inherit: Same as first input
  Wind Shear Model : aerolibwind2/Wind Shear Model  units=Metric (MKS)  phase=Category C - Terminal Flight Phase  W_20=1  Wdeg=0
  vt : Sqrt  SaturateOnIntegerOverflow=on
  windVelocity : Outport  Unit=m/s
  windOmega : Outport  Port=2  Unit=rad/second
  wires:
  [Altitude] -> Dryden Wind Turbulence Model (Continuous (+q +r))/1
  [DCM_be] -> Dryden Wind Turbulence Model (Continuous (+q +r))/3
  [DCM_be] -> Wind Shear Model/2
  DCM_be/1 -> [DCM_be]
  [Altitude] -> Wind Shear Model/1
  Altitude/1 -> [Altitude]
  [Airspeed] -> Discrete Wind Gust Model/1
  vt/1 -> [Airspeed]  "Airspeed"
  Dot Product/1 -> vt/1
  Dryden Wind Turbulence Model (Continuous (+q +r))/2 -> windOmega/1  "WindAngularRates"
  [Airspeed] -> Dryden Wind Turbulence Model (Continuous (+q +r))/2  "Airspeed"
  Sum/1 -> windVelocity/1  "WindVelocity"
  Discrete Wind Gust Model/1 -> Sum/3
  Dryden Wind Turbulence Model (Continuous (+q +r))/1 -> Sum/2
  Wind Shear Model/1 -> Sum/1
  Ve/1 -> Dot Product/2, Dot Product/1

== system mainV02_12/FCS/Slider ==

== system mainV02_12/FCS/Slider1 ==

== system mainV02_12/FCS/Slider2 ==

== system mainV02_12/FCS/Slider3 ==

== system mainV02_12/FCS/Slider4 ==

== system mainV02_12/FCS/Slider5 ==

== system mainV02_12/FCS/Slider6 ==

== system mainV02_12/FCS/Slider7 ==

== system mainV02_12/FCS/Slider8 ==

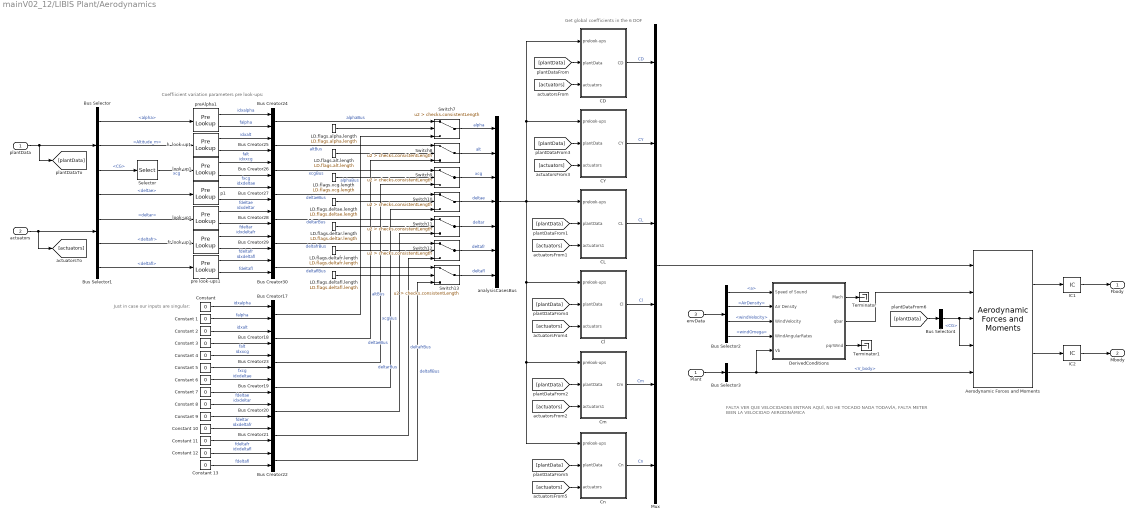
== system mainV02_12/LIBIS Plant/Aerodynamics ==
  note: FALTA VER QUE VELOCIDADES ENTRAN AQUÏ,
      | NO HE TOCADO NADA TODAVÍA, FALTA METER
      | BIEN LA VELOCIDAD AERODINÁMICA
  note: Just in case our inputs are singular:
  note: Get global coefficients in the 6 DOF
  note: Coeffiicient variation parameters pre look-ups:
  plantData : Inport
  actuators : Inport  Port=2
  envData : Inport  Port=3
  " look-up1" : PreLookup  BreakpointsData=LD.xcg  BeginIndexSearchUsingPreviousIndexResult=on  IndexDataTypeStr=int32  FractionDataTypeStr=double
  "Aerodynamic Forces and Moments " : aerolibadyn/Aerodynamic Forces and Moments   inputAxes=Stability  outputForceAxes=Body  outputMomentAxes=Body  S=LD.sref  b=LD.blref  cbar=LD.cbar
  Bus Creator17 : BusCreator  Inputs='idxalpha','falpha'  OutDataTypeStr=Bus: alphaBus  NonVirtualBus=on
  Bus Creator18 : BusCreator  Inputs='idxalt','falt'  OutDataTypeStr=Bus: altBus  NonVirtualBus=on
  Bus Creator19 : BusCreator  Inputs='idxdeltae','fdeltae'  OutDataTypeStr=Bus: deltaeBus  NonVirtualBus=on
  Bus Creator20 : BusCreator  Inputs='idxdeltar','fdeltar'  OutDataTypeStr=Bus: deltarBus  NonVirtualBus=on
  Bus Creator21 : BusCreator  Inputs='idxdeltafr','fdeltafr'  OutDataTypeStr=Bus: deltafrBus  NonVirtualBus=on
  Bus Creator22 : BusCreator  Inputs='idxdeltafl','fdeltafl'  OutDataTypeStr=Bus: deltaflBus  NonVirtualBus=on
  Bus Creator23 : BusCreator  Inputs='idxxcg','fxcg'  OutDataTypeStr=Bus: xcgBus  NonVirtualBus=on
  Bus Creator24 : BusCreator  Inputs='idxalpha','falpha'  OutDataTypeStr=Bus: alphaBus  NonVirtualBus=on
  Bus Creator25 : BusCreator  Inputs='idxalt','falt'  OutDataTypeStr=Bus: altBus  NonVirtualBus=on
  Bus Creator26 : BusCreator  Inputs='idxxcg','fxcg'  OutDataTypeStr=Bus: xcgBus  NonVirtualBus=on
  Bus Creator27 : BusCreator  Inputs='idxdeltae','fdeltae'  OutDataTypeStr=Bus: deltaeBus  NonVirtualBus=on
  Bus Creator28 : BusCreator  Inputs='idxdeltar','fdeltar'  OutDataTypeStr=Bus: deltarBus  NonVirtualBus=on
  Bus Creator29 : BusCreator  Inputs='idxdeltafr','fdeltafr'  OutDataTypeStr=Bus: deltafrBus  NonVirtualBus=on
  Bus Creator30 : BusCreator  Inputs='idxdeltafl','fdeltafl'  OutDataTypeStr=Bus: deltaflBus  NonVirtualBus=on
  Bus Selector : BusSelector  OutputSignals=alpha,LLA.Altitude_m,CG
  Bus Selector1 : BusSelector  OutputSignals=deltae,deltar,deltafr,deltafl
  Bus Selector2 : BusSelector  OutputSignals=a,AirDensity,windVelocity,windOmega
  Bus Selector3 : BusSelector  OutputSignals=V_body
  Bus Selector4 : BusSelector  OutputSignals=CG
  CD : Subsystem
  CL : Subsystem
  CY : Subsystem
  Cl : Subsystem
  Cm : Subsystem
  Cn : Subsystem
  Constant {,2,4,6,8,10,12} (7 alike) : Constant  Value=0  OutDataTypeStr=int32
  Constant {1,3,5,7,9,11,13} (7 alike) : Constant  Value=0
  DerivedConditions : Subsystem
  IC1 : InitialCondition  Value=[0 0 0]
  IC2 : InitialCondition  Value=[0 0 0]
  LD.flags.alpha.length : Constant  Value=LD.flags.alpha.length
  LD.flags.alt.length : Constant  Value=LD.flags.alt.length
  LD.flags.deltae.length : Constant  Value=LD.flags.deltae.length
  LD.flags.deltafl.length : Constant  Value=LD.flags.deltafl.length
  LD.flags.deltafr.length : Constant  Value=LD.flags.deltafr.length
  LD.flags.deltar.length : Constant  Value=LD.flags.deltar.length
  LD.flags.xcg.length : Constant  Value=LD.flags.xcg.length
  Mux : Mux  Inputs=6
  "Plant " : InportShadow
  Selector : Selector  InputPortWidth=3  IndexOptions=Index vector (dialog)  Indices=[1 ]  OutputSizes=1
  Switch{7..13} (7 alike) : Switch  Criteria=u2 > Threshold  Threshold=checks.consistentLength
  Terminator : Terminator
  Terminator1 : Terminator
  analysisCasesBus : BusCreator  Inputs='alpha','alt','xcg','deltae','deltar','deltafr','deltafl'  OutDataTypeStr=Bus: analysisCasesBus  NonVirtualBus=on
  fr look-up1 : PreLookup  BreakpointsData=LD.deltafr  BeginIndexSearchUsingPreviousIndexResult=on  IndexDataTypeStr=int32  FractionDataTypeStr=double
  h  look-up1 : PreLookup  BreakpointsData=LD.alt  BeginIndexSearchUsingPreviousIndexResult=on  IndexDataTypeStr=int32  FractionDataTypeStr=double
  look-up1 : PreLookup  BreakpointsData=LD.deltar  BeginIndexSearchUsingPreviousIndexResult=on  IndexDataTypeStr=int32  FractionDataTypeStr=double
  p1 : PreLookup  BreakpointsData=LD.deltae  BeginIndexSearchUsingPreviousIndexResult=on  IndexDataTypeStr=int32  FractionDataTypeStr=double
  pre look-ups1 : PreLookup  BreakpointsData=LD.deltafl  BeginIndexSearchUsingPreviousIndexResult=on  IndexDataTypeStr=int32  FractionDataTypeStr=double
  preAlpha1 : PreLookup  BreakpointsData=LD.alpha  BeginIndexSearchUsingPreviousIndexResult=on  IndexDataTypeStr=int32  FractionDataTypeStr=double
  Fbody : Outport  Unit=N
  Mbody : Outport  Port=2  Unit=N*m
  wires:
  plantData/1 -> Bus Selector/1, [plantData]
  preAlpha1/2 -> Bus Creator24/2  "falpha"
  preAlpha1/1 -> Bus Creator24/1  "idxalpha"
  h  look-up1/2 -> Bus Creator25/2  "falt"
  h  look-up1/1 -> Bus Creator25/1  "idxalt"
  " look-up1"/1 -> Bus Creator26/1  "idxxcg"
  " look-up1"/2 -> Bus Creator26/2  "fxcg"
  p1/2 -> Bus Creator27/2  "fdeltae"
  p1/1 -> Bus Creator27/1  "idxdeltae"
  look-up1/2 -> Bus Creator28/2  "fdeltar"
  look-up1/1 -> Bus Creator28/1  "idxdeltar"
  fr look-up1/2 -> Bus Creator29/2  "fdeltafr"
  fr look-up1/1 -> Bus Creator29/1  "idxdeltafr"
  pre look-ups1/1 -> Bus Creator30/1  "idxdeltafl"
  pre look-ups1/2 -> Bus Creator30/2  "fdeltafl"
  LD.flags.alpha.length/1 -> Switch7/2
  Bus Creator24/1 -> Switch7/1  "alphaBus"
  LD.flags.alt.length/1 -> Switch8/2
  Bus Creator25/1 -> Switch8/1  "altBus"
  LD.flags.xcg.length/1 -> Switch9/2
  Bus Creator26/1 -> Switch9/1  "xcgBus"
  LD.flags.deltae.length/1 -> Switch10/2
  Bus Creator27/1 -> Switch10/1  "deltaeBus"
  LD.flags.deltar.length/1 -> Switch11/2
  Bus Creator28/1 -> Switch11/1  "deltarBus"
  LD.flags.deltafr.length/1 -> Switch12/2
  Bus Creator29/1 -> Switch12/1  "deltafrBus"
  LD.flags.deltafl.length/1 -> Switch13/2
  Bus Creator30/1 -> Switch13/1  "deltaflBus"
  Bus Creator17/1 -> Switch7/3  "alphaBus"
  Bus Creator18/1 -> Switch8/3  "altBus"
  Bus Creator23/1 -> Switch9/3  "xcgBus"
  Bus Creator19/1 -> Switch10/3  "deltaeBus"
  Bus Creator20/1 -> Switch11/3  "deltarBus"
  Bus Creator21/1 -> Switch12/3  "deltafrBus"
  Bus Creator22/1 -> Switch13/3  "deltaflBus"
  Switch7/1 -> analysisCasesBus/1  "alpha"
  Switch8/1 -> analysisCasesBus/2  "alt"
  Switch9/1 -> analysisCasesBus/3  "xcg"
  Switch10/1 -> analysisCasesBus/4  "deltae"
  Switch11/1 -> analysisCasesBus/5  "deltar"
  Switch12/1 -> analysisCasesBus/6  "deltafr"
  Switch13/1 -> analysisCasesBus/7  "deltafl"
  Constant 1/1 -> Bus Creator17/2  "falpha"
  "Constant "/1 -> Bus Creator17/1  "idxalpha"
  Constant 3/1 -> Bus Creator18/2  "falt"
  Constant 2/1 -> Bus Creator18/1  "idxalt"
  Constant 4/1 -> Bus Creator23/1  "idxxcg"
  Constant 5/1 -> Bus Creator23/2  "fxcg"
  Constant 7/1 -> Bus Creator19/2  "fdeltae"
  Constant 6/1 -> Bus Creator19/1  "idxdeltae"
  Constant 9/1 -> Bus Creator20/2  "fdeltar"
  Constant 8/1 -> Bus Creator20/1  "idxdeltar"
  Constant 11/1 -> Bus Creator21/2  "fdeltafr"
  Constant 10/1 -> Bus Creator21/1  "idxdeltafr"
  Constant 12/1 -> Bus Creator22/1  "idxdeltafl"
  Constant 13/1 -> Bus Creator22/2  "fdeltafl"
  analysisCasesBus/1 -> Cl/1(prelook-ups), Cm/1(prelook-ups), Cn/1(prelook-ups), CD/1(prelook-ups), CY/1(prelook-ups), CL/1(prelook-ups)
  Bus Selector/1 -> preAlpha1/1  "<alpha>"
  Bus Selector/2 -> h  look-up1/1  "<Altitude_m>"
  Bus Selector/3 -> Selector/1  "<CG>"
  Selector/1 -> " look-up1"/1  "xcg"
  actuators/1 -> [actuators], Bus Selector1/1
  Bus Selector1/1 -> p1/1  "<deltae>"
  Bus Selector1/2 -> look-up1/1  "<deltar>"
  Bus Selector1/3 -> fr look-up1/1  "<deltafr>"
  Bus Selector1/4 -> pre look-ups1/1  "<deltafl>"
  [plantData] -> CD/2(plantData)
  [actuators] -> CD/3(actuators)
  [plantData] -> CL/2(plantData)
  [plantData] -> Cm/2(plantData)
  [plantData] -> CY/2(plantData)
  [actuators] -> CY/3(actuators)
  [plantData] -> Cl/2(plantData)
  [actuators] -> Cl/3(actuators)
  [plantData] -> Cn/2(plantData)
  [actuators] -> Cn/3(actuators)
  Cn/1(Cn) -> Mux/6  "Cn"
  Cl/1(Cl) -> Mux/4  "Cl"
  CL/1(CL) -> Mux/3  "CL"
  CY/1(CY) -> Mux/2  "CY"
  CD/1(CD) -> Mux/1  "CD"
  Cm/1(Cm) -> Mux/5  "Cm"
  Mux/1 -> "Aerodynamic Forces and Moments "/1
  "Aerodynamic Forces and Moments "/1 -> IC1/1
  "Aerodynamic Forces and Moments "/2 -> IC2/1
  envData/1 -> Bus Selector2/1
  Bus Selector2/1 -> DerivedConditions/1(Speed of Sound)  "<a>"
  Bus Selector2/2 -> DerivedConditions/2(Air Density)  "<AirDensity>"
  Bus Selector2/3 -> DerivedConditions/3(WindVelocity)  "<windVelocity>"
  Bus Selector2/4 -> DerivedConditions/4(WindAngularRates)  "<windOmega>"
  "Plant "/1 -> Bus Selector3/1
  Bus Selector3/1 -> DerivedConditions/5(Vb), "Aerodynamic Forces and Moments "/5  "<V_body>"
  DerivedConditions/1(Mach) -> Terminator/1
  DerivedConditions/3("pqrWind ") -> Terminator1/1
  DerivedConditions/2(qbar) -> "Aerodynamic Forces and Moments "/2
  [plantData] -> Bus Selector4/1
  Bus Selector4/1 -> "Aerodynamic Forces and Moments "/4, "Aerodynamic Forces and Moments "/3  "<CG>"
  [actuators] -> CL/3(actuators1)
  [actuators] -> Cm/3(actuators1)
  IC1/1 -> Fbody/1
  IC2/1 -> Mbody/1

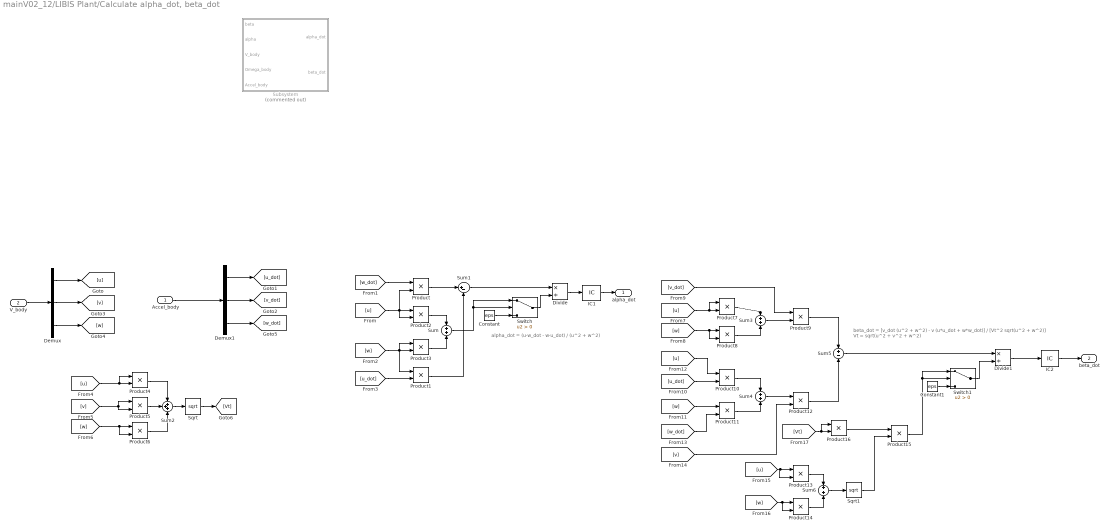
== system mainV02_12/LIBIS Plant/Calculate alpha_dot, beta_dot ==
  note: beta_dot = [v_dot (u^2 + w^2) - v (u*u_dot + w*w_dot)] / [Vt^2 sqrt(u^2 + w^2)]
      | Vt = sqrt(u^2 + v^2 + w^2)
  note: alpha_dot = (u·w_dot - w·u_dot) / (u^2 + w^2)
  Accel_body : Inport  Unit=meter/s^2
  V_body : Inport  Port=2  Unit=meter/s
  Constant : Constant  Value=eps
  Constant1 : Constant  Value=eps
  Demux : Demux  Outputs=3
  Demux1 : Demux  Outputs=3
  Divide : Product  Inputs=*/
  Divide1 : Product  Inputs=*/
  IC1 : InitialCondition  Value=0
  IC2 : InitialCondition  Value=0
  Product{,1..16} (17 alike) : Product
  Sqrt : Sqrt  SaturateOnIntegerOverflow=on
  Sqrt1 : Sqrt  SaturateOnIntegerOverflow=on
  Subsystem : Subsystem  Commented=on
  Sum{,3..4,6} (4 alike) : Sum  Inputs=+|+
  Sum1 : Sum  Inputs=|+-
  Sum2 : Sum  Inputs=+++
  Sum5 : Sum  Inputs=+|-
  Switch : Switch  Criteria=u2 > Threshold
  Switch1 : Switch  Criteria=u2 > Threshold
  alpha_dot : Outport  Unit=rad/s
  beta_dot : Outport  Port=2
  wires:
  V_body/1 -> Demux/1
  Demux/1 -> [u]
  Demux/2 -> [v]
  Demux/3 -> [w]
  [w_dot] -> Product/1
  [u] -> Product/2, Product2/2, Product2/1
  [w] -> Product3/1, Product3/2, Product1/1
  [u_dot] -> Product1/2
  Product2/1 -> Sum/1
  Product3/1 -> Sum/2
  Product/1 -> Sum1/1
  Product1/1 -> Sum1/2
  Sum1/1 -> Divide/1
  [u] -> Product4/1, Product4/2
  [w] -> Product6/2, Product6/1
  [v] -> Product5/1, Product5/2
  Product4/1 -> Sum2/1
  Product6/1 -> Sum2/3
  Product5/1 -> Sum2/2
  Sum2/1 -> Sqrt/1
  Sqrt/1 -> [Vt]
  [u] -> Product7/1, Product7/2
  [w] -> Product8/2, Product8/1
  Product7/1 -> Sum3/1
  Product8/1 -> Sum3/2
  Sum3/1 -> Product9/2
  [v_dot] -> Product9/1
  [u_dot] -> Product10/2
  [w] -> Product11/1
  Product10/1 -> Sum4/1
  Product11/1 -> Sum4/2
  Sum4/1 -> Product12/1
  [u] -> Product10/1
  [w_dot] -> Product11/2
  [v] -> Product12/2
  Product9/1 -> Sum5/1
  Product12/1 -> Sum5/2
  Sum5/1 -> Divide1/1
  Product13/1 -> Sum6/1
  Product14/1 -> Sum6/2
  [u] -> Product13/2, Product13/1
  [w] -> Product14/2, Product14/1
  [Vt] -> Product16/1, Product16/2
  Product16/1 -> Product15/1
  Sum6/1 -> Sqrt1/1
  Sqrt1/1 -> Product15/2
  Demux1/1 -> [u_dot]
  Demux1/2 -> [v_dot]
  Demux1/3 -> [w_dot]
  Accel_body/1 -> Demux1/1
  Divide/1 -> IC1/1
  Switch/1 -> Divide/2
  Sum/1 -> Switch/2, Switch/1
  Constant/1 -> Switch/3
  Divide1/1 -> IC2/1
  Switch1/1 -> Divide1/2
  Product15/1 -> Switch1/2, Switch1/1
  Constant1/1 -> Switch1/3
  IC1/1 -> alpha_dot/1
  IC2/1 -> beta_dot/1

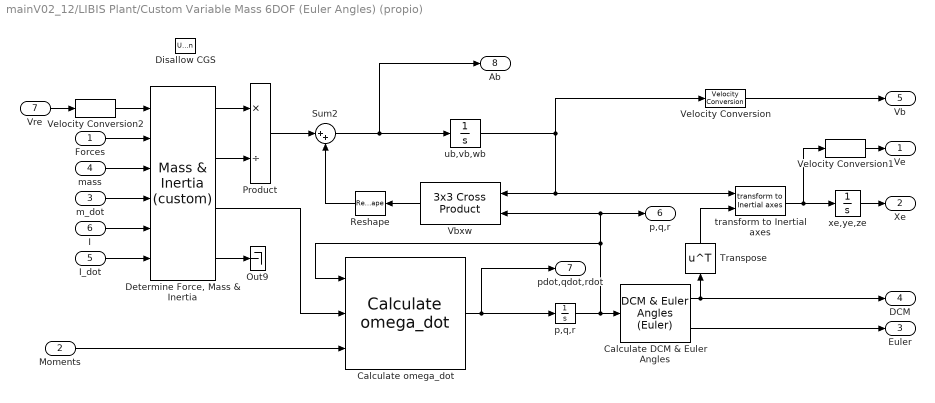
== system mainV02_12/LIBIS Plant/Custom Variable Mass 6DOF (Euler Angles) (propio) ==
  Forces : Inport  Unit=N  PortDimensions=3
  Moments : Inport  Port=2  Unit=N*m  PortDimensions=3
  m_dot : Inport  Port=3  Unit=kg/s
  mass : Inport  Port=4  Unit=kg
  I_dot : Inport  Port=5  Unit=kg*m^2/s  PortDimensions=[3 3]
  I : Inport  Port=6  Unit=kg*m^2  PortDimensions=[3 3]
  Vre : Inport  Port=7  Unit=m/s
  Calculate DCM & Euler Angles : aerolib6dofsys/DCM & Euler Angles (Euler)  SystemSampleTime=-1
  Calculate omega_dot : aerolib6dofsys/Calculate omega_dot  SystemSampleTime=-1
  "Determine Force, Mass & Inertia" : aerolib6dofsys/Mass & Inertia (custom)  SystemSampleTime=-1
  Disallow CGS : UnitConfiguration  UnitSystemsStr=English,SI,SI (extended)  AllowAllUnitSystems=off
  Out9 : Terminator
  Product : Product  Inputs=*/  SaturateOnIntegerOverflow=on  OutDataTypeStr=Inherit: Same as first input
  Reshape : Reshape  OutputDimensions=""
  Sum2 : Sum  Inputs=|++  SaturateOnIntegerOverflow=on
  Transpose : Math  Operator=transpose  SaturateOnIntegerOverflow=on
  Vbxw : aerolibutil/3x3 Cross Product
  Velocity Conversion : aerolib6dof2/6DOF (Euler Angles)/Velocity Conversion
  Velocity Conversion1 : aerolib6dof2/6DOF (Euler Angles)/Velocity Conversion1
  Velocity Conversion2 : aerolib6dof2/6DOF (Euler Angles)/Velocity Conversion2
  "p,q,r " : Integrator  InitialCondition=pm_0
  "transform to Inertial axes " : aerolib6dof2/6DOF (Euler Angles)/transform to Inertial axes   SystemSampleTime=-1
  ub,vb,wb : Integrator  InitialCondition=Vm_0
  xe,ye,ze : Integrator  InitialCondition=xme_0  UpperSaturationLimit=[inf, inf, initialValues.href]  LowerSaturationLimit=[-inf, -inf, -inf]
  Ve : Outport  Unit=m/s
  Xe : Outport  Port=2  Unit=m
  Euler : Outport  Port=3  Unit=rad
  DCM : Outport  Port=4  Unit=1
  Vb : Outport  Port=5  Unit=m/s
  p,q,r : Outport  Port=6  Unit=rad/s
  pdot,qdot,rdot : Outport  Port=7  Unit=rad/s^2
  Ab : Outport  Port=8  Unit=m/s^2  PortDimensions=3
  wires:
  Velocity Conversion1/1 -> Ve/1
  "Determine Force, Mass & Inertia"/2 -> Product/2
  Vre/1 -> Velocity Conversion2/1
  Calculate DCM & Euler Angles/1 -> DCM/1, Transpose/1
  Transpose/1 -> "transform to Inertial axes "/2
  Calculate DCM & Euler Angles/2 -> Euler/1
  "Determine Force, Mass & Inertia"/4 -> Out9/1
  "p,q,r "/1 -> Calculate DCM & Euler Angles/1, p,q,r/1, Vbxw/2, Calculate omega_dot/1
  xe,ye,ze/1 -> Xe/1
  Velocity Conversion/1 -> Vb/1
  I_dot/1 -> "Determine Force, Mass & Inertia"/6
  "transform to Inertial axes "/1 -> Velocity Conversion1/1, xe,ye,ze/1
  mass/1 -> "Determine Force, Mass & Inertia"/3
  Velocity Conversion2/1 -> "Determine Force, Mass & Inertia"/1
  "Determine Force, Mass & Inertia"/1 -> Product/1
  Forces/1 -> "Determine Force, Mass & Inertia"/2
  Moments/1 -> Calculate omega_dot/3
  Product/1 -> Sum2/1
  m_dot/1 -> "Determine Force, Mass & Inertia"/4
  ub,vb,wb/1 -> Vbxw/1, "transform to Inertial axes "/1, Velocity Conversion/1
  "Determine Force, Mass & Inertia"/3 -> Calculate omega_dot/2
  I/1 -> "Determine Force, Mass & Inertia"/5
  Sum2/1 -> Ab/1, ub,vb,wb/1
  Calculate omega_dot/1 -> pdot,qdot,rdot/1, "p,q,r "/1
  Vbxw/1 -> Reshape/1
  Reshape/1 -> Sum2/2
